simulink model "Contol_PID_OPC"  (R2013a)
settings: Solver=ode45  StartTime=0.0  StopTime=4500  RelTol=1e-3
InitFcn:
  | load('Kp.mat')
  | load('Kd.mat')
  | load('Ki.mat')
values from neighbouring files (symbols this model uses):
  Kd = -2.1308168557    [Kd.mat]
  Ki = 0.22046236166    [Kd.mat]
  Kp = 4.86450734815    [Kd.mat]
libraries: opclib x3, simulink x1
settings Model: Creator=alvares  LastModifiedBy=Cristhian Ivan

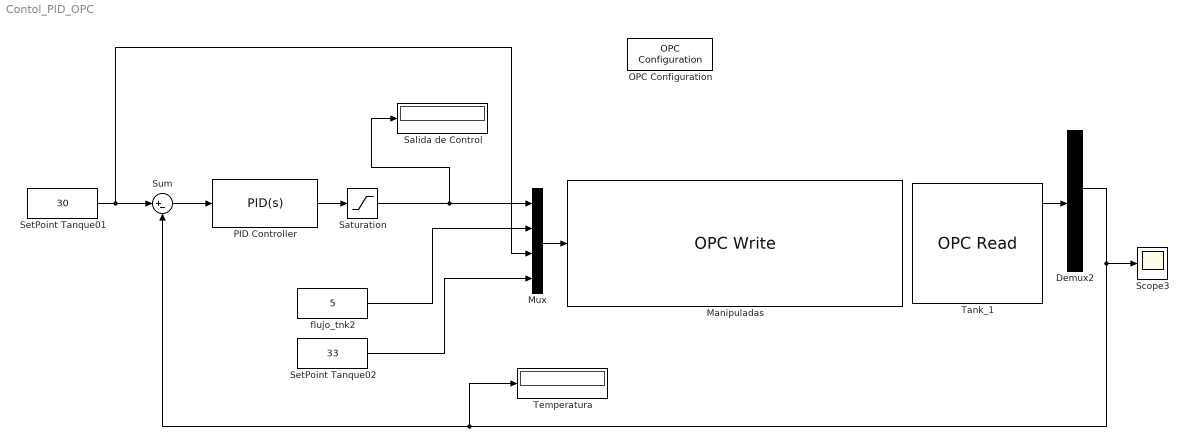
== system Contol_PID_OPC ==
  Demux2 : Demux  Outputs=6
  Manipuladas : opclib/OPC Write  serverHost=164.41.17.129  serverID=Smar.DfiOleServer.0  itemIDs=TY-31_PID1.OUT.VALUE, FY-32_PID1.OUT.VALUE, TY-31_PID1.SP.VALUE, FY-32_PID1.SP.VALUE  writeMode=Synchronous  updateRate=0.5
  Mux : Mux
  OPC Configuration : opclib/OPC Configuration  opcServers=164.41.17.129/Smar.DfiOleServer.0/10  errMissingItems=Error  errReadWrite=Warn  errShutdown=Error  errRTViolation=Warn  rtEnable=on  speedup=1  showLatency=off  beingUsed=on
  PID Controller : simulink/Continuous/PID Controller  Controller=PID  TimeDomain=Continuous-time  SampleTime=1  IntegratorMethod=Forward Euler  FilterMethod=Forward Euler  Form=Parallel  P=Kp  I=Ki  D=Kd  N=100  InitialConditionSource=internal  InitialConditionForIntegrator=0  InitialConditionForFilter=0  ExternalReset=none  LimitOutput=off  UpperSaturationLimit=inf  LowerSaturationLimit=-inf  LinearizeAsGain=on  AntiWindupMode=none  Kb=1  TrackingMode=off  Kt=1  PParamMin=[]  PParamMax=[]  IParamMin=[]  IParamMax=[]  DParamMin=[]  DParamMax=[]  NParamMin=[]  NParamMax=[]  KbParamMin=[]  KbParamMax=[]  KtParamMin=[]  KtParamMax=[]  POutMin=[]  POutMax=[]  IOutMin=[]  IOutMax=[]  DOutMin=[]  DOutMax=[]  NOutMin=[]  NOutMax=[]  KbOutMin=[]  KbOutMax=[]  KtOutMin=[]  KtOutMax=[]  IntegratorOutMin=[]  IntegratorOutMax=[]  FilterOutMin=[]  FilterOutMax=[]  SumOutMin=[]  SumOutMax=[]  SumI1OutMin=[]  SumI1OutMax=[]  SumI2OutMin=[]  SumI2OutMax=[]  SumI3OutMin=[]  SumI3OutMax=[]  SumDOutMin=[]  SumDOutMax=[]  SaturationOutMin=[]  SaturationOutMax=[]  IntegratorContinuousStateAttributes=''  IntegratorStateMustResolveToSignalObject=off  IntegratorRTWStateStorageClass=Auto  FilterContinuousStateAttributes=''  FilterStateMustResolveToSignalObject=off  FilterRTWStateStorageClass=Auto
  Salida de Control : Display
  Saturation : Saturate  UpperLimit=100  LowerLimit=-100  ZeroCross=off
  Scope3 : Scope
      settings: YMin=44.0345  YMax=44.0455  SaveName=PID_Proba_01
  SetPoint Tanque01 : Constant  Value=30
  SetPoint Tanque02 : Constant  Value=33
  Sum : Sum  Inputs=|+-
  Tank_1 : opclib/OPC Read  serverHost=164.41.17.129  serverID=Smar.DfiOleServer.0  itemIDs=TY-31_PID1.OUT.VALUE, FIT-31_AI1.OUT, TIT-31_AI1.OUT.VALUE, FY-31_AO1.OUT.VALUE, TY-31_PID1.SP.VALUE, TY-31_AO1.OUT.VALUE  readMode=Synchronous (cache)  dataType=single  updateRate=0.001  showQual=on  showTS=on  tsMode=Seconds since start
  Temperatura : Display
  flujo_tnk2 : Constant  Value=5
  wires:
  Mux/1 -> Manipuladas/1
  Demux2/3 -> Temperatura/1, Sum/2, Scope3/1
  Tank_1/1 -> Demux2/1
  SetPoint Tanque02/1 -> Mux/4
  flujo_tnk2/1 -> Mux/2
  PID Controller/1 -> Saturation/1
  Sum/1 -> PID Controller/1
  Saturation/1 -> Salida de Control/1, Mux/1
  SetPoint Tanque01/1 -> Mux/3, Sum/1
